simulink model "ENV_old"  (R2024b)
settings: Solver=FixedStepDiscrete  StartTime=0.0  StopTime=1  FixedStep=0.001  RelTol=1e-3  EnableMultiTasking=on
libraries: stm32blockslib x84, canmsglib x40, stm32f4xxblockslib x8, simulink x7
(part 3 of 4)

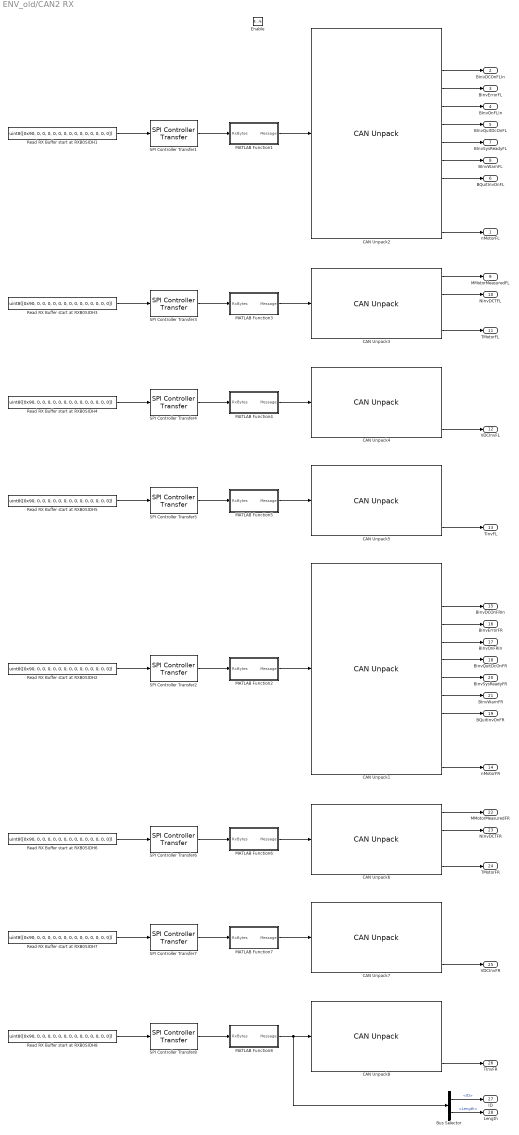
== system ENV_old/CAN2 RX ==
  Enable : EnablePort
  Bus Selector : BusSelector  OutputSignals=ID,Length
  CAN Unpack1 : canmsglib/CAN Unpack  CANdbFile=C:\Users\Will\Desktop\OBR\Embedded\VCUSTM32\Controls\CAN\Inverters\26.06.18_CAN2.dbc  MsgList=INV4_Send_1  MsgName=INV4_Send_1  MsgIDType=Standard (11-bit identifier)  MsgIdentifier=658  MsgLength=8  SignalInfo={'AMK_bDerating','47','1','LE','unsigned','Standard','0','1','0','0','1';'AMK_bReserve','32','8','LE','signed','Standard','0','1','0','-128','127';'BInvDCOnFRIn','44','1','LE','unsigned','Standard','0','1','0','0','1';'BInvErrorFR','41','1','LE','unsigned','Standard','0','1','0','0','1';'BInvOnFRIn','46','1','LE','unsigned','Standard','0','1','0','0','1';'BInvQuitDcOnFR','43','1','LE','unsigned','Standard','0','1','0','0','1';'BInvSysReadyFR','40','1','LE','unsigned','Standard','0','1','0','0','1';'BInvWarnFR','42','1','LE','unsigned','Standard','0','1','0','0','1';'BQuitInvOnFR','45','1','LE','unsigned','Standard','0','1','0','0','1';'Checksum','16','16','LE','unsigned','Standard','0','1','0','0','65535';'Message_Counter','0','16','LE','unsigned','Standard','0','1','0','0','65535';'nMotorFR','48','16','LE','signed','Standard','0','1','0','-32768','32767'}  IDPort=off  TimestampPort=off  ErrorPort=off  RemotePort=off  LengthPort=off  StatusPort=off  ApplyMinMax=off
      settings: LibrarySourceBlock=stmutilitieslib/CAN Unpack  DataFormat=CANdb specified signals
  CAN Unpack2 : canmsglib/CAN Unpack  CANdbFile=C:\Users\Will\Desktop\OBR\Embedded\VCUSTM32\Controls\CAN\Inverters\26.06.18_CAN2.dbc  MsgList=INV2_Send_1  MsgName=INV2_Send_1  MsgIDType=Standard (11-bit identifier)  MsgIdentifier=657  MsgLength=8  SignalInfo={'AMK_bDerating','47','1','LE','unsigned','Standard','0','1','0','0','1';'AMK_bReserve','32','8','LE','signed','Standard','0','1','0','-128','127';'BInvDCOnFLIn','44','1','LE','unsigned','Standard','0','1','0','0','1';'BInvErrorFL','41','1','LE','unsigned','Standard','0','1','0','0','1';'BInvOnFLIn','46','1','LE','unsigned','Standard','0','1','0','0','1';'BInvQuitDcOnFL','43','1','LE','unsigned','Standard','0','1','0','0','1';'BInvSysReadyFL','40','1','LE','unsigned','Standard','0','1','0','0','1';'BInvWarnFL','42','1','LE','unsigned','Standard','0','1','0','0','1';'BQuitInvOnFL','45','1','LE','unsigned','Standard','0','1','0','0','1';'Checksum','16','16','LE','unsigned','Standard','0','1','0','0','65535';'Message_Counter','0','16','LE','unsigned','Standard','0','1','0','0','65535';'nMotorFL','48','16','LE','signed','Standard','0','1','0','-32768','32767'}  IDPort=off  TimestampPort=off  ErrorPort=off  RemotePort=off  LengthPort=off  StatusPort=off  ApplyMinMax=off
      settings: LibrarySourceBlock=stmutilitieslib/CAN Unpack  DataFormat=CANdb specified signals
  CAN Unpack3 : canmsglib/CAN Unpack  CANdbFile=C:\Users\Will\Desktop\OBR\Embedded\VCUSTM32\Controls\CAN\Inverters\26.06.18_CAN2.dbc  MsgList=INV2_Send_2  MsgName=INV2_Send_2  MsgIDType=Standard (11-bit identifier)  MsgIdentifier=659  MsgLength=8  SignalInfo={'MMotorMeasuredFL','16','16','LE','signed','Standard','0','1','0','-32768','32767';'NInvDTCFL','32','16','LE','signed','Standard','0','1','0','-32768','32767';'NInvErrorInfoFL1','48','16','LE','signed','Standard','0','1','0','-32768','32767';'TMotorFL','0','16','LE','signed','Standard','0','0.1','0','-3276.8','3276.7'}  IDPort=off  TimestampPort=off  ErrorPort=off  RemotePort=off  LengthPort=off  StatusPort=off  ApplyMinMax=off
      settings: LibrarySourceBlock=stmutilitieslib/CAN Unpack  DataFormat=CANdb specified signals
  CAN Unpack4 : canmsglib/CAN Unpack  CANdbFile=C:\Users\Will\Desktop\OBR\Embedded\VCUSTM32\Controls\CAN\Inverters\26.06.18_CAN2.dbc  MsgList=INV2_Send_3  MsgName=INV2_Send_3  MsgIDType=Standard (11-bit identifier)  MsgIdentifier=661  MsgLength=8  SignalInfo={'NInvErrorInfoFL2','0','16','LE','signed','Standard','0','1','0','-32768','32767';'NInvErrorInfoFL3','16','16','LE','signed','Standard','0','1','0','-32768','32767';'Raw_Torque_Current','32','16','LE','signed','Standard','0','1','0','-32768','32767';'VDCInvFL','48','16','LE','signed','Standard','0','1','0','-32768','32767'}  IDPort=off  TimestampPort=off  ErrorPort=off  RemotePort=off  LengthPort=off  StatusPort=off  ApplyMinMax=off
      settings: LibrarySourceBlock=stmutilitieslib/CAN Unpack  DataFormat=CANdb specified signals
  CAN Unpack5 : canmsglib/CAN Unpack  CANdbFile=C:\Users\Will\Desktop\OBR\Embedded\VCUSTM32\Controls\CAN\Inverters\26.06.18_CAN2.dbc  MsgList=INV2_Send_4  MsgName=INV2_Send_4  MsgIDType=Standard (11-bit identifier)  MsgIdentifier=663  MsgLength=8  SignalInfo={'Converter_Peak_Current','32','16','LE','signed','Standard','0','1','0','-32768','32767';'Motor_Nomial_Current_IN','48','16','LE','signed','Standard','0','1','0','-32768','32767';'Motor_Peak_Current','16','16','LE','signed','Standard','0','1','0','-32768','32767';'TInvFL','0','16','LE','signed','Standard','0','0.1','0','-3276.8','3276.7'}  IDPort=off  TimestampPort=off  ErrorPort=off  RemotePort=off  LengthPort=off  StatusPort=off  ApplyMinMax=off
      settings: LibrarySourceBlock=stmutilitieslib/CAN Unpack  DataFormat=CANdb specified signals
  CAN Unpack6 : canmsglib/CAN Unpack  CANdbFile=C:\Users\Will\Desktop\OBR\Embedded\VCUSTM32\Controls\CAN\Inverters\26.06.18_CAN2.dbc  MsgList=INV4_Send_2  MsgName=INV4_Send_2  MsgIDType=Standard (11-bit identifier)  MsgIdentifier=660  MsgLength=8  SignalInfo={'MMotorMeasuredFR','16','16','LE','signed','Standard','0','1','0','-32768','32767';'NInvDTCFR','32','16','LE','signed','Standard','0','1','0','-32768','32767';'NInvErrorInfoFR1','48','16','LE','signed','Standard','0','1','0','-32768','32767';'TMotorFR','0','16','LE','signed','Standard','0','0.1','0','-3276.8','3276.7'}  IDPort=off  TimestampPort=off  ErrorPort=off  RemotePort=off  LengthPort=off  StatusPort=off  ApplyMinMax=off
      settings: LibrarySourceBlock=stmutilitieslib/CAN Unpack  DataFormat=CANdb specified signals
  CAN Unpack7 : canmsglib/CAN Unpack  CANdbFile=C:\Users\Will\Desktop\OBR\Embedded\VCUSTM32\Controls\CAN\Inverters\26.06.18_CAN2.dbc  MsgList=INV4_Send_3  MsgName=INV4_Send_3  MsgIDType=Standard (11-bit identifier)  MsgIdentifier=662  MsgLength=8  SignalInfo={'NInvErrorInfoFR2','0','16','LE','signed','Standard','0','1','0','-32768','32767';'NInvErrorInfoFR3','16','16','LE','signed','Standard','0','1','0','-32768','32767';'Raw_Torque_Current','32','16','LE','signed','Standard','0','1','0','-32768','32767';'VDCInvFR','48','16','LE','signed','Standard','0','1','0','-32768','32767'}  IDPort=off  TimestampPort=off  ErrorPort=off  RemotePort=off  LengthPort=off  StatusPort=off  ApplyMinMax=off
      settings: LibrarySourceBlock=stmutilitieslib/CAN Unpack  DataFormat=CANdb specified signals
  CAN Unpack8 : canmsglib/CAN Unpack  CANdbFile=C:\Users\Will\Desktop\OBR\Embedded\VCUSTM32\Controls\CAN\Inverters\26.06.18_CAN2.dbc  MsgList=INV4_Send_4  MsgName=INV4_Send_4  MsgIDType=Standard (11-bit identifier)  MsgIdentifier=664  MsgLength=8  SignalInfo={'Converter_Peak_Current','32','16','LE','signed','Standard','0','1','0','-32768','32767';'Motor_Nomial_Current_IN','48','16','LE','signed','Standard','0','1','0','-32768','32767';'Motor_Peak_Current','16','16','LE','signed','Standard','0','1','0','-32768','32767';'TInvFR','0','16','LE','signed','Standard','0','0.1','0','-3276.8','3276.7'}  IDPort=off  TimestampPort=off  ErrorPort=off  RemotePort=off  LengthPort=off  StatusPort=off  ApplyMinMax=off
      settings: LibrarySourceBlock=stmutilitieslib/CAN Unpack  DataFormat=CANdb specified signals
  MATLAB Function1 : MATLAB Function  TreatAsAtomicUnit=on
  MATLAB Function2 : MATLAB Function  TreatAsAtomicUnit=on
  MATLAB Function3 : MATLAB Function  TreatAsAtomicUnit=on
  MATLAB Function4 : MATLAB Function  TreatAsAtomicUnit=on
  MATLAB Function5 : MATLAB Function  TreatAsAtomicUnit=on
  MATLAB Function6 : MATLAB Function  TreatAsAtomicUnit=on
  MATLAB Function7 : MATLAB Function  TreatAsAtomicUnit=on
  MATLAB Function8 : MATLAB Function  TreatAsAtomicUnit=on
  Read RX Buffer start at RXB0SIDH{1..8} (8 alike) : Constant  Value=uint8([0x90, 0, 0, 0, 0, 0, 0, 0, 0, 0, 0, 0, 0, 0, 0])
  SPI Controller Transfer{1..8} (8 alike) : stm32blockslib/SPI Controller Transfer  Priority=1  SPIModuleSelect=SPI1  ClockPolarity=Low  ClockPhase=1 Edge  SPIModule=uint32(0)  Mode=Master  BusSpeed=uint32(1000000)  FirstBitToTransfer=Most significant bit (MSB)  ClockMode=0  BlockFunction=Transfer  EnableRegisterAddress=off  RegisterAddress=0  OutputDataType=uint8  OutputDataLength=1  OutputStatus=off  BlockingMode=on  Timeout=0.01  DataBits=8  UseCustomSSPin=Explicit GPIO calls  ActiveLowSSPin=Active low  Port_Select=GPIOC  Pin=10
      settings: LibrarySourceBlock=stm32h7xxblockslib/SPI Controller Transfer
  nMotorFL : Outport  OutDataTypeStr=double
  BInvDCOnFLIn : Outport  Port=2  OutDataTypeStr=boolean
  BInvErrorFL : Outport  Port=3  OutDataTypeStr=boolean
  BInvOnFLIn : Outport  Port=4  OutDataTypeStr=boolean
  BInvQuitDcOnFL : Outport  Port=5  OutDataTypeStr=boolean
  BQuitInvOnFL : Outport  Port=6  OutDataTypeStr=boolean
  BInvSysReadyFL : Outport  Port=7  OutDataTypeStr=boolean
  BInvWarnFL : Outport  Port=8  OutDataTypeStr=boolean
  MMotorMeasuredFL : Outport  Port=9  OutDataTypeStr=double
  NInvDCTFL : Outport  Port=10  OutDataTypeStr=double
  TMotorFL : Outport  Port=11  OutDataTypeStr=double
  VDCInvFL : Outport  Port=12  OutDataTypeStr=double
  TInvFL : Outport  Port=13  OutDataTypeStr=double
  nMotorFR : Outport  Port=14  OutDataTypeStr=double
  BInvDCOnFRIn : Outport  Port=15  OutDataTypeStr=boolean
  BInvErrorFR : Outport  Port=16  OutDataTypeStr=boolean
  BInvOnFRIn : Outport  Port=17  OutDataTypeStr=boolean
  BInvQuitDcOnFR : Outport  Port=18  OutDataTypeStr=boolean
  BQuitInvOnFR : Outport  Port=19  OutDataTypeStr=boolean
  BInvSysReadyFR : Outport  Port=20  OutDataTypeStr=boolean
  BInvWarnFR : Outport  Port=21  OutDataTypeStr=boolean
  MMotorMeasuredFR : Outport  Port=22  OutDataTypeStr=double
  NInvDCTFR : Outport  Port=23  OutDataTypeStr=double
  TMotorFR : Outport  Port=24  OutDataTypeStr=double
  VDCInvFR : Outport  Port=25  OutDataTypeStr=double
  TInvFR : Outport  Port=26  OutDataTypeStr=double
  ID : Outport  Port=27
  Length : Outport  Port=28
  wires:
  Read RX Buffer start at RXB0SIDH1/1 -> SPI Controller Transfer1/1
  SPI Controller Transfer1/1 -> MATLAB Function1/1(RxBytes)
  MATLAB Function1/1(Message) -> CAN Unpack2/1
  CAN Unpack2/3 -> BInvDCOnFLIn/1
  CAN Unpack2/4 -> BInvErrorFL/1
  CAN Unpack2/5 -> BInvOnFLIn/1
  CAN Unpack2/6 -> BInvQuitDcOnFL/1
  CAN Unpack2/9 -> BQuitInvOnFL/1
  CAN Unpack2/8 -> BInvWarnFL/1
  CAN Unpack2/7 -> BInvSysReadyFL/1
  CAN Unpack2/12 -> nMotorFL/1
  CAN Unpack3/4 -> TMotorFL/1
  MATLAB Function3/1(Message) -> CAN Unpack3/1
  SPI Controller Transfer3/1 -> MATLAB Function3/1(RxBytes)
  Read RX Buffer start at RXB0SIDH3/1 -> SPI Controller Transfer3/1
  CAN Unpack3/1 -> MMotorMeasuredFL/1
  CAN Unpack3/2 -> NInvDCTFL/1
  CAN Unpack4/4 -> VDCInvFL/1
  SPI Controller Transfer4/1 -> MATLAB Function4/1(RxBytes)
  MATLAB Function4/1(Message) -> CAN Unpack4/1
  Read RX Buffer start at RXB0SIDH4/1 -> SPI Controller Transfer4/1
  SPI Controller Transfer5/1 -> MATLAB Function5/1(RxBytes)
  CAN Unpack5/4 -> TInvFL/1
  Read RX Buffer start at RXB0SIDH5/1 -> SPI Controller Transfer5/1
  MATLAB Function5/1(Message) -> CAN Unpack5/1
  MATLAB Function8/1(Message) -> Bus Selector/1, CAN Unpack8/1
  Bus Selector/2 -> Length/1  "<Length>"
  Bus Selector/1 -> ID/1  "<ID>"
  CAN Unpack1/6 -> BInvQuitDcOnFR/1
  CAN Unpack1/3 -> BInvDCOnFRIn/1
  CAN Unpack6/4 -> TMotorFR/1
  CAN Unpack1/5 -> BInvOnFRIn/1
  SPI Controller Transfer2/1 -> MATLAB Function2/1(RxBytes)
  MATLAB Function2/1(Message) -> CAN Unpack1/1
  SPI Controller Transfer8/1 -> MATLAB Function8/1(RxBytes)
  CAN Unpack1/8 -> BInvWarnFR/1
  CAN Unpack6/1 -> MMotorMeasuredFR/1
  CAN Unpack1/12 -> nMotorFR/1
  CAN Unpack1/4 -> BInvErrorFR/1
  CAN Unpack1/7 -> BInvSysReadyFR/1
  CAN Unpack1/9 -> BQuitInvOnFR/1
  Read RX Buffer start at RXB0SIDH2/1 -> SPI Controller Transfer2/1
  SPI Controller Transfer7/1 -> MATLAB Function7/1(RxBytes)
  Read RX Buffer start at RXB0SIDH8/1 -> SPI Controller Transfer8/1
  MATLAB Function6/1(Message) -> CAN Unpack6/1
  Read RX Buffer start at RXB0SIDH7/1 -> SPI Controller Transfer7/1
  CAN Unpack6/2 -> NInvDCTFR/1
  SPI Controller Transfer6/1 -> MATLAB Function6/1(RxBytes)
  MATLAB Function7/1(Message) -> CAN Unpack7/1
  Read RX Buffer start at RXB0SIDH6/1 -> SPI Controller Transfer6/1
  CAN Unpack7/4 -> VDCInvFR/1
  CAN Unpack8/4 -> TInvFR/1

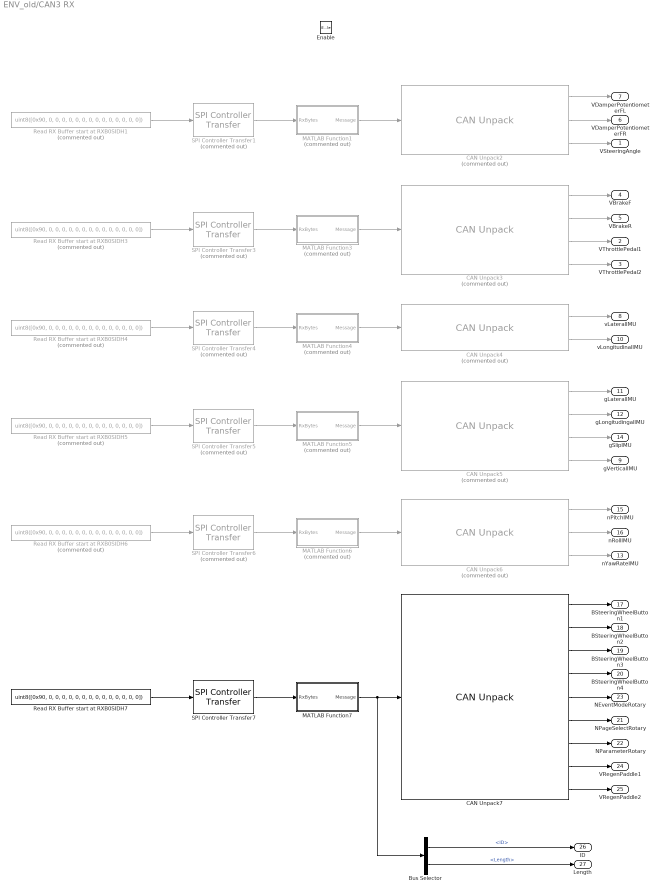
== system ENV_old/CAN3 RX ==
  Enable : EnablePort
  Bus Selector : BusSelector  OutputSignals=ID,Length
  CAN Unpack2 : canmsglib/CAN Unpack  Commented=on  CANdbFile=C:\Users\oxbro\Documents\STM32CustomProjects\VCUSTM32\OBR26_Controls_30-7-26\CAN\CAN3\CAN3_03.08.26.dbc  MsgList=(none)  MsgName=DDU7_SteerDamper  MsgIDType=Standard (11-bit identifier)  MsgIdentifier=257  MsgLength=8  SignalInfo={'VDamperPotentiometerFL','16','13','LE','unsigned','Standard','0','1','0','0','8191';'VDamperPotentiometerFR','29','13','LE','unsigned','Standard','0','1','0','0','8191';'VSteeringAngle','0','13','LE','unsigned','Standard','0','1','0','0','8191'}  IDPort=off  TimestampPort=off  ErrorPort=off  RemotePort=off  LengthPort=off  StatusPort=off  ApplyMinMax=off
      settings: LibrarySourceBlock=stmutilitieslib/CAN Unpack  DataFormat=CANdb specified signals
  CAN Unpack3 : canmsglib/CAN Unpack  Commented=on  CANdbFile=C:\Users\oxbro\Documents\STM32CustomProjects\VCUSTM32\OBR26_Controls_30-7-26\CAN\CAN3\CAN3_03.08.26.dbc  MsgList=(none)  MsgName=DDU7_ThrBrake  MsgIDType=Standard (11-bit identifier)  MsgIdentifier=256  MsgLength=8  SignalInfo={'VBrakeF','0','16','LE','unsigned','Standard','0','1','0','0','3276.75';'VBrakeR','16','16','LE','unsigned','Standard','0','1','0','0','65535';'VThrottlePedal1','32','16','LE','unsigned','Standard','0','1','0','0','65535';'VThrottlePedal2','48','16','LE','unsigned','Standard','0','1','0','0','65535'}  IDPort=off  TimestampPort=off  ErrorPort=off  RemotePort=off  LengthPort=off  StatusPort=off  ApplyMinMax=off
      settings: LibrarySourceBlock=stmutilitieslib/CAN Unpack  DataFormat=CANdb specified signals
  CAN Unpack4 : canmsglib/CAN Unpack  Commented=on  CANdbFile=C:\Users\oxbro\Documents\STM32CustomProjects\VCUSTM32\OBR26_Controls_30-7-26\CAN\CAN3\CAN3_03.08.26.dbc  MsgList=(none)  MsgName=IMU_0x604  MsgIDType=Standard (11-bit identifier)  MsgIdentifier=1540  MsgLength=8  SignalInfo={'vLateralIMU','16','16','LE','signed','Standard','0','0.01','0','-327.68','327.67';'vLongitudinalIMU','0','16','LE','signed','Standard','0','0.01','0','-327.68','327.67'}  IDPort=off  TimestampPort=off  ErrorPort=off  RemotePort=off  LengthPort=off  StatusPort=off  ApplyMinMax=off
      settings: LibrarySourceBlock=stmutilitieslib/CAN Unpack  DataFormat=CANdb specified signals
  CAN Unpack5 : canmsglib/CAN Unpack  Commented=on  CANdbFile=C:\Users\oxbro\Documents\STM32CustomProjects\VCUSTM32\OBR26_Controls_30-7-26\CAN\CAN3\CAN3_03.08.26.dbc  MsgList=(none)  MsgName=IMU_0x606  MsgIDType=Standard (11-bit identifier)  MsgIdentifier=1542  MsgLength=8  SignalInfo={'gLateralIMU','16','16','LE','signed','Standard','0','0.01','0','-327.68','327.67';'gLongitudinalIMU','0','16','LE','signed','Standard','0','0.01','0','-327.68','327.67';'gSlipIMU','48','16','LE','signed','Standard','0','0.01','0','-327.68','327.67';'gVerticalIMU','32','16','LE','signed','Standard','0','0.01','0','-327.68','327.67'}  IDPort=off  TimestampPort=off  ErrorPort=off  RemotePort=off  LengthPort=off  StatusPort=off  ApplyMinMax=off
      settings: LibrarySourceBlock=stmutilitieslib/CAN Unpack  DataFormat=CANdb specified signals
  CAN Unpack6 : canmsglib/CAN Unpack  Commented=on  CANdbFile=C:\Users\oxbro\Documents\STM32CustomProjects\VCUSTM32\OBR26_Controls_30-7-26\CAN\CAN3\CAN3_03.08.26.dbc  MsgList=(none)  MsgName=IMU_0x609  MsgIDType=Standard (11-bit identifier)  MsgIdentifier=1545  MsgLength=8  SignalInfo={'nPitchIMU','16','16','LE','signed','Standard','0','0.01','0','-327.68','327.67';'nRollIMU','0','16','LE','signed','Standard','0','0.01','0','-327.68','327.67';'nYawRateIMU','32','16','LE','signed','Standard','0','0.01','0','-327.68','327.67'}  IDPort=off  TimestampPort=off  ErrorPort=off  RemotePort=off  LengthPort=off  StatusPort=off  ApplyMinMax=off
      settings: LibrarySourceBlock=stmutilitieslib/CAN Unpack  DataFormat=CANdb specified signals
  CAN Unpack7 : canmsglib/CAN Unpack  CANdbFile=C:\Users\oxbro\Documents\STM32CustomProjects\VCUSTM32\OBR26_Controls_30-7-26\CAN\CAN3\CAN3_03.08.26.dbc  MsgList=STW_0x1FB  MsgName=STW_0x1FB  MsgIDType=Standard (11-bit identifier)  MsgIdentifier=507  MsgLength=6  SignalInfo={'BSteeringWheelButton1','0','1','LE','unsigned','Standard','0','1','0','0','1';'BSteeringWheelButton2','1','1','LE','unsigned','Standard','0','1','0','0','1';'BSteeringWheelButton3','2','1','LE','unsigned','Standard','0','1','0','0','1';'BSteeringWheelButton4','3','1','LE','unsigned','Standard','0','1','0','0','1';'NEventModeRotary','20','8','LE','unsigned','Standard','0','1','1','1','16';'NPageSelectRotary','4','8','LE','unsigned','Standard','0','1','1','1','16';'NParameterRotary','12','8','LE','unsigned','Standard','0','1','1','1','16';'VRegenPaddle1','28','8','LE','unsigned','Standard','0','0.0129','0','0','3.2895';'VRegenPaddle2','36','8','LE','unsigned','Standard','0','0.0129','0','0','3.2895'}  IDPort=off  TimestampPort=off  ErrorPort=off  RemotePort=off  LengthPort=off  StatusPort=off  ApplyMinMax=off
      settings: LibrarySourceBlock=stmutilitieslib/CAN Unpack  DataFormat=CANdb specified signals
  MATLAB Function1 : MATLAB Function  Commented=on  TreatAsAtomicUnit=on
  MATLAB Function3 : MATLAB Function  Commented=on  TreatAsAtomicUnit=on
  MATLAB Function4 : MATLAB Function  Commented=on  TreatAsAtomicUnit=on
  MATLAB Function5 : MATLAB Function  Commented=on  TreatAsAtomicUnit=on
  MATLAB Function6 : MATLAB Function  Commented=on  TreatAsAtomicUnit=on
  MATLAB Function7 : MATLAB Function  TreatAsAtomicUnit=on
  Read RX Buffer start at RXB0SIDH{1,3..6} (5 alike) : Constant  Commented=on  Value=uint8([0x90, 0, 0, 0, 0, 0, 0, 0, 0, 0, 0, 0, 0, 0, 0])
  Read RX Buffer start at RXB0SIDH7 : Constant  Value=uint8([0x90, 0, 0, 0, 0, 0, 0, 0, 0, 0, 0, 0, 0, 0, 0])
  SPI Controller Transfer{1,3..6} (5 alike) : stm32blockslib/SPI Controller Transfer  Priority=1  Commented=on  SPIModuleSelect=SPI1  ClockPolarity=Low  ClockPhase=1 Edge  SPIModule=uint32(0)  Mode=Master  BusSpeed=uint32(1000000)  FirstBitToTransfer=Most significant bit (MSB)  ClockMode=0  BlockFunction=Transfer  EnableRegisterAddress=off  RegisterAddress=0  OutputDataType=uint8  OutputDataLength=1  OutputStatus=off  BlockingMode=on  Timeout=0.01  DataBits=8  UseCustomSSPin=Explicit GPIO calls  ActiveLowSSPin=Active low  Port_Select=GPIOA  Pin=1
      settings: LibrarySourceBlock=stm32h7xxblockslib/SPI Controller Transfer
  SPI Controller Transfer7 : stm32blockslib/SPI Controller Transfer  Priority=1  SPIModuleSelect=SPI1  ClockPolarity=Low  ClockPhase=1 Edge  SPIModule=uint32(0)  Mode=Master  BusSpeed=uint32(1000000)  FirstBitToTransfer=Most significant bit (MSB)  ClockMode=0  BlockFunction=Transfer  EnableRegisterAddress=off  RegisterAddress=0  OutputDataType=uint8  OutputDataLength=1  OutputStatus=off  BlockingMode=on  Timeout=0.01  DataBits=8  UseCustomSSPin=Explicit GPIO calls  ActiveLowSSPin=Active low  Port_Select=GPIOA  Pin=1
      settings: LibrarySourceBlock=stm32h7xxblockslib/SPI Controller Transfer
  VSteeringAngle : Outport  OutDataTypeStr=double
  VThrottlePedal1 : Outport  Port=2  OutDataTypeStr=double
  VThrottlePedal2 : Outport  Port=3  OutDataTypeStr=double
  VBrakeF : Outport  Port=4  OutDataTypeStr=double
  VBrakeR : Outport  Port=5  OutDataTypeStr=double
  VDamperPotentiometerFR : Outport  Port=6  OutDataTypeStr=double
  VDamperPotentiometerFL : Outport  Port=7  OutDataTypeStr=double
  vLateralIMU : Outport  Port=8  OutDataTypeStr=double
  gVerticalIMU : Outport  Port=9  OutDataTypeStr=double
  vLongitudinalIMU : Outport  Port=10  OutDataTypeStr=double
  gLateralIMU : Outport  Port=11  OutDataTypeStr=double
  gLongitudingalIMU : Outport  Port=12  OutDataTypeStr=double
  nYawRateIMU : Outport  Port=13  OutDataTypeStr=double
  gSlipIMU : Outport  Port=14  OutDataTypeStr=double
  nPitchIMU : Outport  Port=15  OutDataTypeStr=double
  nRollIMU : Outport  Port=16  OutDataTypeStr=double
  BSteeringWheelButton1 : Outport  Port=17  OutDataTypeStr=boolean
  BSteeringWheelButton2 : Outport  Port=18  OutDataTypeStr=boolean
  BSteeringWheelButton3 : Outport  Port=19  OutDataTypeStr=boolean
  BSteeringWheelButton4 : Outport  Port=20  OutDataTypeStr=boolean
  NPageSelectRotary : Outport  Port=21  OutDataTypeStr=double
  NParameterRotary : Outport  Port=22  OutDataTypeStr=double
  NEventModeRotary : Outport  Port=23  OutDataTypeStr=double
  VRegenPaddle1 : Outport  Port=24  OutDataTypeStr=double
  VRegenPaddle2 : Outport  Port=25  OutDataTypeStr=double
  ID : Outport  Port=26
  Length : Outport  Port=27
  wires:
  Bus Selector/1 -> ID/1  "<ID>"
  Bus Selector/2 -> Length/1  "<Length>"
  CAN Unpack4/1 -> vLateralIMU/1
  CAN Unpack7/5 -> NEventModeRotary/1
  CAN Unpack7/3 -> BSteeringWheelButton3/1
  CAN Unpack2/1 -> VDamperPotentiometerFL/1
  CAN Unpack2/2 -> VDamperPotentiometerFR/1
  CAN Unpack5/4 -> gVerticalIMU/1
  CAN Unpack3/3 -> VThrottlePedal1/1
  CAN Unpack2/3 -> VSteeringAngle/1
  CAN Unpack6/2 -> nRollIMU/1
  CAN Unpack7/6 -> NPageSelectRotary/1
  CAN Unpack7/1 -> BSteeringWheelButton1/1
  CAN Unpack6/3 -> nYawRateIMU/1
  CAN Unpack3/1 -> VBrakeF/1
  CAN Unpack5/2 -> gLongitudingalIMU/1
  CAN Unpack7/9 -> VRegenPaddle2/1
  CAN Unpack7/7 -> NParameterRotary/1
  CAN Unpack7/2 -> BSteeringWheelButton2/1
  CAN Unpack3/4 -> VThrottlePedal2/1
  CAN Unpack3/2 -> VBrakeR/1
  CAN Unpack7/8 -> VRegenPaddle1/1
  CAN Unpack6/1 -> nPitchIMU/1
  CAN Unpack5/3 -> gSlipIMU/1
  CAN Unpack7/4 -> BSteeringWheelButton4/1
  CAN Unpack4/2 -> vLongitudinalIMU/1
  CAN Unpack5/1 -> gLateralIMU/1
  Read RX Buffer start at RXB0SIDH1/1 -> SPI Controller Transfer1/1
  SPI Controller Transfer1/1 -> MATLAB Function1/1(RxBytes)
  MATLAB Function1/1(Message) -> CAN Unpack2/1
  MATLAB Function3/1(Message) -> CAN Unpack3/1
  Read RX Buffer start at RXB0SIDH3/1 -> SPI Controller Transfer3/1
  SPI Controller Transfer3/1 -> MATLAB Function3/1(RxBytes)
  MATLAB Function4/1(Message) -> CAN Unpack4/1
  Read RX Buffer start at RXB0SIDH4/1 -> SPI Controller Transfer4/1
  SPI Controller Transfer4/1 -> MATLAB Function4/1(RxBytes)
  Read RX Buffer start at RXB0SIDH5/1 -> SPI Controller Transfer5/1
  SPI Controller Transfer5/1 -> MATLAB Function5/1(RxBytes)
  MATLAB Function5/1(Message) -> CAN Unpack5/1
  Read RX Buffer start at RXB0SIDH6/1 -> SPI Controller Transfer6/1
  SPI Controller Transfer6/1 -> MATLAB Function6/1(RxBytes)
  MATLAB Function6/1(Message) -> CAN Unpack6/1
  Read RX Buffer start at RXB0SIDH7/1 -> SPI Controller Transfer7/1
  SPI Controller Transfer7/1 -> MATLAB Function7/1(RxBytes)
  MATLAB Function7/1(Message) -> Bus Selector/1, CAN Unpack7/1

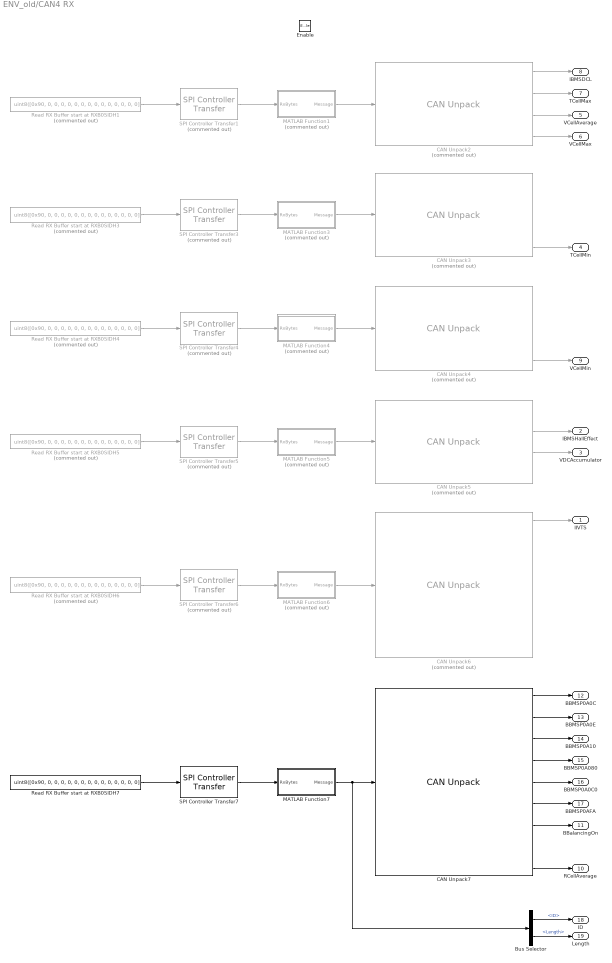
== system ENV_old/CAN4 RX ==
  Enable : EnablePort
  Bus Selector : BusSelector  OutputSignals=ID,Length
  CAN Unpack2 : canmsglib/CAN Unpack  Commented=on  CANdbFile=C:\Users\Will\Desktop\OBR\Embedded\VCUSTM32\Controls\CAN\BMS\26.06.18_CAN4.dbc  MsgList=MSGID_0X6B2  MsgName=MSGID_0X6B2  MsgIDType=Standard (11-bit identifier)  MsgIdentifier=1714  MsgLength=8  SignalInfo={'IBMSDCL','48','16','LE','unsigned','Standard','0','1','0','0','65535';'TCellMax','40','16','BE','signed','Standard','0','1','0','80','32767';'VCellAverage','8','16','BE','unsigned','Standard','0','1e-08','0','0','0.00065535';'VCellMax','24','16','BE','unsigned','Standard','0','0.0001','0','0','6.5535'}  IDPort=off  TimestampPort=off  ErrorPort=off  RemotePort=off  LengthPort=off  StatusPort=off  ApplyMinMax=off
      settings: LibrarySourceBlock=stmutilitieslib/CAN Unpack  DataFormat=CANdb specified signals
  CAN Unpack3 : canmsglib/CAN Unpack  Commented=on  CANdbFile=C:\Users\Will\Desktop\OBR\Embedded\VCUSTM32\Controls\CAN\BMS\26.06.18_CAN4.dbc  MsgList=MSGID_0X6B1  MsgName=MSGID_0X6B1  MsgIDType=Standard (11-bit identifier)  MsgIdentifier=1713  MsgLength=8  SignalInfo={'DTC_Flags_1','16','16','LE','unsigned','Standard','0','1','0','0','65535';'DTC_Flags_2','40','16','BE','unsigned','Standard','0','1','0','0','65535';'Pack_SOC','8','16','BE','unsigned','Standard','0','0.5','0','0','32767.5';'TCellMin','56','16','BE','signed','Standard','0','1','0','80','32767'}  IDPort=off  TimestampPort=off  ErrorPort=off  RemotePort=off  LengthPort=off  StatusPort=off  ApplyMinMax=off
      settings: LibrarySourceBlock=stmutilitieslib/CAN Unpack  DataFormat=CANdb specified signals
  CAN Unpack4 : canmsglib/CAN Unpack  Commented=on  CANdbFile=C:\Users\Will\Desktop\OBR\Embedded\VCUSTM32\Controls\CAN\BMS\26.06.18_CAN4.dbc  MsgList=MSGID_0X6B3  MsgName=MSGID_0X6B3  MsgIDType=Standard (11-bit identifier)  MsgIdentifier=1715  MsgLength=8  SignalInfo={'High_Cell_Resistance','8','16','BE','unsigned','Standard','0','0.01','0','0','655';'Maximum_Cell_Voltage','40','16','BE','unsigned','Standard','0','0.0001','0','0','6.5535';'Minimum_Cell_Voltage','56','16','BE','unsigned','Standard','0','0.0001','0','0','6.5535';'VCellMin','24','16','BE','unsigned','Standard','0','0.0001','0','0','6.5535'}  IDPort=off  TimestampPort=off  ErrorPort=off  RemotePort=off  LengthPort=off  StatusPort=off  ApplyMinMax=off
      settings: LibrarySourceBlock=stmutilitieslib/CAN Unpack  DataFormat=CANdb specified signals
  CAN Unpack5 : canmsglib/CAN Unpack  Commented=on  CANdbFile=C:\Users\Will\Desktop\OBR\Embedded\VCUSTM32\Controls\CAN\BMS\26.06.18_CAN4.dbc  MsgList=MSGID_0X6B0  MsgName=MSGID_0X6B0  MsgIDType=Standard (11-bit identifier)  MsgIdentifier=1712  MsgLength=8  SignalInfo={'CRC_Checksum','48','16','LE','unsigned','Standard','0','1','0','0','65535';'IBMSHallEffect','32','16','LE','signed','Standard','0','1','0','32767','32767';'VDCAccumulator','16','16','LE','unsigned','Standard','0','1','0','0','65535';'VDCAccumulator_NOT','8','16','BE','unsigned','Standard','0','0.1','0','0','6553.5'}  IDPort=off  TimestampPort=off  ErrorPort=off  RemotePort=off  LengthPort=off  StatusPort=off  ApplyMinMax=off
      settings: LibrarySourceBlock=stmutilitieslib/CAN Unpack  DataFormat=CANdb specified signals
  CAN Unpack6 : canmsglib/CAN Unpack  Commented=on  CANdbFile=C:\Users\Will\Desktop\OBR\Embedded\VCUSTM32\Controls\CAN\BMS\26.06.18_CAN4.dbc  MsgList=IVT_Msg_Result_I  MsgName=IVT_Msg_Result_I  MsgIDType=Standard (11-bit identifier)  MsgIdentifier=1313  MsgLength=6  SignalInfo={'IIVTS','40','32','BE','signed','Standard','0','1','0','-2147483648','2147483647';'IVT_ID_Result_I','0','8','BE','unsigned','Standard','0','1','0','0','255';'IVT_MsgCount_Result_I','8','4','BE','unsigned','Standard','0','1','0','0','15';'IVT_Result_I_Channel_Error','13','1','BE','unsigned','Standard','0','1','0','0','1';'IVT_Result_I_Measurement_Error','14','1','BE','unsigned','Standard','0','1','0','0','1';'IVT_Result_I_OCS','12','1','BE','unsigned','Standard','0','1','0','0','1';'IVT_Result_I_System_Error','15','1','BE','unsigned','Standard','0','1','0','0','1'}  IDPort=off  TimestampPort=off  ErrorPort=off  RemotePort=off  LengthPort=off  StatusPort=off  ApplyMinMax=off
      settings: LibrarySourceBlock=stmutilitieslib/CAN Unpack  DataFormat=CANdb specified signals
  CAN Unpack7 : canmsglib/CAN Unpack  CANdbFile=C:\Users\Will\Desktop\OBR\Embedded\VCUSTM32\Controls\CAN\BMS\26.06.18_CAN4.dbc  MsgList=MSGID_0X6B4  MsgName=MSGID_0X6B4  MsgIDType=Standard (11-bit identifier)  MsgIdentifier=1716  MsgLength=8  SignalInfo={'BBMSP0A0C','33','1','LE','unsigned','Standard','0','1','0','0','1';'BBMSP0A0E','34','1','LE','unsigned','Standard','0','1','0','0','1';'BBMSP0A10','35','1','LE','unsigned','Standard','0','1','0','0','1';'BBMSP0A80','36','1','LE','unsigned','Standard','0','1','0','0','1';'BBMSP0AC0','37','1','LE','unsigned','Standard','0','1','0','0','1';'BBMSP0AFA','38','1','LE','unsigned','Standard','0','1','0','0','1';'BBalancingOn','32','1','LE','unsigned','Standard','0','1','0','0','1';'Blank','56','8','LE','unsigned','Standard','0','1','0','0','255';'RCellAverage','8','16','BE','unsigned','Standard','0','0.01','0','0','655'}  IDPort=off  TimestampPort=off  ErrorPort=off  RemotePort=off  LengthPort=off  StatusPort=off  ApplyMinMax=off
      settings: LibrarySourceBlock=stmutilitieslib/CAN Unpack  DataFormat=CANdb specified signals
  MATLAB Function1 : MATLAB Function  Commented=on  TreatAsAtomicUnit=on
  MATLAB Function3 : MATLAB Function  Commented=on  TreatAsAtomicUnit=on
  MATLAB Function4 : MATLAB Function  Commented=on  TreatAsAtomicUnit=on
  MATLAB Function5 : MATLAB Function  Commented=on  TreatAsAtomicUnit=on
  MATLAB Function6 : MATLAB Function  Commented=on  TreatAsAtomicUnit=on
  MATLAB Function7 : MATLAB Function  TreatAsAtomicUnit=on
  Read RX Buffer start at RXB0SIDH{1,3..6} (5 alike) : Constant  Commented=on  Value=uint8([0x90, 0, 0, 0, 0, 0, 0, 0, 0, 0, 0, 0, 0, 0, 0])
  Read RX Buffer start at RXB0SIDH7 : Constant  Value=uint8([0x90, 0, 0, 0, 0, 0, 0, 0, 0, 0, 0, 0, 0, 0, 0])
  SPI Controller Transfer{1,3..6} (5 alike) : stm32blockslib/SPI Controller Transfer  Priority=1  Commented=on  SPIModuleSelect=SPI1  ClockPolarity=Low  ClockPhase=1 Edge  SPIModule=uint32(0)  Mode=Master  BusSpeed=uint32(1000000)  FirstBitToTransfer=Most significant bit (MSB)  ClockMode=0  BlockFunction=Transfer  EnableRegisterAddress=off  RegisterAddress=0  OutputDataType=uint8  OutputDataLength=1  OutputStatus=off  BlockingMode=on  Timeout=0.01  DataBits=8  UseCustomSSPin=Explicit GPIO calls  ActiveLowSSPin=Active low  Port_Select=GPIOC  Pin=5
      settings: LibrarySourceBlock=stm32h7xxblockslib/SPI Controller Transfer
  SPI Controller Transfer7 : stm32blockslib/SPI Controller Transfer  Priority=1  SPIModuleSelect=SPI1  ClockPolarity=Low  ClockPhase=1 Edge  SPIModule=uint32(0)  Mode=Master  BusSpeed=uint32(1000000)  FirstBitToTransfer=Most significant bit (MSB)  ClockMode=0  BlockFunction=Transfer  EnableRegisterAddress=off  RegisterAddress=0  OutputDataType=uint8  OutputDataLength=1  OutputStatus=off  BlockingMode=on  Timeout=0.01  DataBits=8  UseCustomSSPin=Explicit GPIO calls  ActiveLowSSPin=Active low  Port_Select=GPIOC  Pin=5
      settings: LibrarySourceBlock=stm32h7xxblockslib/SPI Controller Transfer
  IIVTS : Outport  OutDataTypeStr=double
  IBMSHallEffect : Outport  Port=2  OutDataTypeStr=double
  VDCAccumulator : Outport  Port=3  OutDataTypeStr=double
  TCellMin : Outport  Port=4  OutDataTypeStr=double
  VCellAverage : Outport  Port=5  OutDataTypeStr=double
  VCellMax : Outport  Port=6  OutDataTypeStr=double
  TCellMax : Outport  Port=7  OutDataTypeStr=double
  IBMSDCL : Outport  Port=8  OutDataTypeStr=double
  VCellMin : Outport  Port=9  OutDataTypeStr=double
  RCellAverage : Outport  Port=10  OutDataTypeStr=double
  BBalancingOn : Outport  Port=11  OutDataTypeStr=boolean
  BBMSP0A0C : Outport  Port=12  OutDataTypeStr=boolean
  BBMSP0A0E : Outport  Port=13  OutDataTypeStr=boolean
  BBMSP0A10 : Outport  Port=14  OutDataTypeStr=boolean
  BBMSP0A080 : Outport  Port=15  OutDataTypeStr=boolean
  BBMSP0A0C0 : Outport  Port=16  OutDataTypeStr=boolean
  BBMSP0AFA : Outport  Port=17  OutDataTypeStr=boolean
  ID : Outport  Port=18
  Length : Outport  Port=19
  wires:
  Bus Selector/1 -> ID/1  "<ID>"
  Bus Selector/2 -> Length/1  "<Length>"
  CAN Unpack2/1 -> IBMSDCL/1
  CAN Unpack2/2 -> TCellMax/1
  CAN Unpack2/3 -> VCellAverage/1
  CAN Unpack5/2 -> IBMSHallEffect/1
  CAN Unpack6/1 -> IIVTS/1
  CAN Unpack5/3 -> VDCAccumulator/1
  Read RX Buffer start at RXB0SIDH1/1 -> SPI Controller Transfer1/1
  SPI Controller Transfer1/1 -> MATLAB Function1/1(RxBytes)
  MATLAB Function1/1(Message) -> CAN Unpack2/1
  MATLAB Function3/1(Message) -> CAN Unpack3/1
  Read RX Buffer start at RXB0SIDH3/1 -> SPI Controller Transfer3/1
  SPI Controller Transfer3/1 -> MATLAB Function3/1(RxBytes)
  MATLAB Function4/1(Message) -> CAN Unpack4/1
  Read RX Buffer start at RXB0SIDH4/1 -> SPI Controller Transfer4/1
  SPI Controller Transfer4/1 -> MATLAB Function4/1(RxBytes)
  Read RX Buffer start at RXB0SIDH5/1 -> SPI Controller Transfer5/1
  SPI Controller Transfer5/1 -> MATLAB Function5/1(RxBytes)
  MATLAB Function5/1(Message) -> CAN Unpack5/1
  Read RX Buffer start at RXB0SIDH6/1 -> SPI Controller Transfer6/1
  SPI Controller Transfer6/1 -> MATLAB Function6/1(RxBytes)
  MATLAB Function6/1(Message) -> CAN Unpack6/1
  Read RX Buffer start at RXB0SIDH7/1 -> SPI Controller Transfer7/1
  SPI Controller Transfer7/1 -> MATLAB Function7/1(RxBytes)
  MATLAB Function7/1(Message) -> Bus Selector/1, CAN Unpack7/1
  CAN Unpack3/4 -> TCellMin/1
  CAN Unpack2/4 -> VCellMax/1
  CAN Unpack4/4 -> VCellMin/1
  CAN Unpack7/2 -> BBMSP0A0E/1
  CAN Unpack7/3 -> BBMSP0A10/1
  CAN Unpack7/1 -> BBMSP0A0C/1
  CAN Unpack7/9 -> RCellAverage/1
  CAN Unpack7/7 -> BBalancingOn/1
  CAN Unpack7/6 -> BBMSP0AFA/1
  CAN Unpack7/5 -> BBMSP0A0C0/1
  CAN Unpack7/4 -> BBMSP0A080/1

== system ENV_old/Initialize CAN1 ==
  Detect Increase : simulink/Logic and Bit Operations/Detect Increase  vinit=0.0  OutDataTypeStr=boolean
  MCPInit : Subsystem  TreatAsAtomicUnit=on
  Step1 : Step
  Step2 : Step
  Unit Delay : UnitDelay  SampleTime=-1  HasFrameUpgradeWarning=on
  MCPInitialized : Outport
  wires:
  Step1/1 -> Detect Increase/1
  Detect Increase/1 -> MCPInit/Enable
  Step2/1 -> Unit Delay/1
  Unit Delay/1 -> MCPInitialized/1

== system ENV_old/Initialize CAN2 ==
  Detect Increase : simulink/Logic and Bit Operations/Detect Increase  vinit=0.0  OutDataTypeStr=boolean
  MCPInit : Subsystem  TreatAsAtomicUnit=on
  Step1 : Step
  Step2 : Step
  Unit Delay : UnitDelay  SampleTime=-1  HasFrameUpgradeWarning=on
  Unit Delay1 : UnitDelay  SampleTime=-1  HasFrameUpgradeWarning=on
  Unit Delay2 : UnitDelay  SampleTime=-1  HasFrameUpgradeWarning=on
  MCPInitialized : Outport
  wires:
  Step1/1 -> Unit Delay1/1
  Detect Increase/1 -> MCPInit/Enable
  Step2/1 -> Unit Delay/1
  Unit Delay/1 -> Unit Delay2/1
  Unit Delay1/1 -> Detect Increase/1
  Unit Delay2/1 -> MCPInitialized/1

== system ENV_old/Initialize CAN3 ==
  Detect Increase : simulink/Logic and Bit Operations/Detect Increase  vinit=0.0  OutDataTypeStr=boolean
  Initialize : Subsystem  TreatAsAtomicUnit=on
  MCPInit : Subsystem  TreatAsAtomicUnit=on
  Step1 : Step
  Step2 : Step
  Unit Delay{1..5} (5 alike) : UnitDelay  SampleTime=-1  HasFrameUpgradeWarning=on
  MCPInitialized : Outport
  wires:
  Initialize/1(MCPInitialized) -> MCPInitialized/1
  Detect Increase/1 -> MCPInit/Enable
  Step1/1 -> Unit Delay3/1
  Step2/1 -> Unit Delay1/1
  Unit Delay3/1 -> Unit Delay4/1
  Unit Delay4/1 -> Detect Increase/1
  Unit Delay1/1 -> Unit Delay2/1
  Unit Delay2/1 -> Unit Delay5/1
  Unit Delay5/1 -> Initialize/Enable

== system ENV_old/Initialize CAN4 ==
  Detect Increase : simulink/Logic and Bit Operations/Detect Increase  vinit=0.0  OutDataTypeStr=boolean
  MCPInit : Subsystem  TreatAsAtomicUnit=on
  Step1 : Step
  Step2 : Step
  Unit Delay{1..7} (7 alike) : UnitDelay  SampleTime=-1  HasFrameUpgradeWarning=on
  MCPInitialized : Outport
  wires:
  Step1/1 -> Unit Delay3/1
  Detect Increase/1 -> MCPInit/Enable
  Step2/1 -> Unit Delay7/1
  Unit Delay3/1 -> Unit Delay1/1
  Unit Delay1/1 -> Unit Delay2/1
  Unit Delay2/1 -> Detect Increase/1
  Unit Delay4/1 -> Unit Delay5/1
  Unit Delay5/1 -> Unit Delay6/1
  Unit Delay6/1 -> MCPInitialized/1
  Unit Delay7/1 -> Unit Delay4/1

== system ENV_old/Subsystem1 ==
  Detect Increase : simulink/Logic and Bit Operations/Detect Increase  vinit=0.0  OutDataTypeStr=boolean
  Initialize : Subsystem  TreatAsAtomicUnit=on
  MCPInit : Subsystem  TreatAsAtomicUnit=on
  Step1 : Step
  Step2 : Step
  Unit Delay : UnitDelay  SampleTime=-1  HasFrameUpgradeWarning=on
  MCPInitialized : Outport
  wires:
  Step1/1 -> Detect Increase/1
  Unit Delay/1 -> Initialize/Enable
  Detect Increase/1 -> MCPInit/Enable
  Step2/1 -> Unit Delay/1
  Initialize/1(MCPInitialized) -> MCPInitialized/1

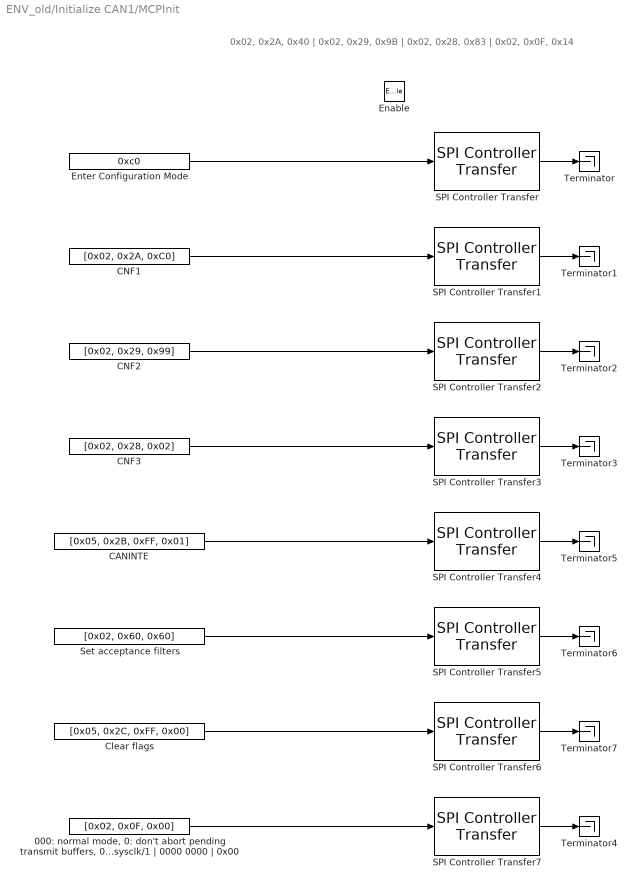
== system ENV_old/Initialize CAN1/MCPInit ==
  note: 0x02, 0x2A, 0x40 | 0x02, 0x29, 0x9B | 0x02, 0x28, 0x83 | 0x02, 0x0F, 0x14
  Enable : EnablePort
  " 000: normal mode, 0: don't abort pending transmit buffers, 0: one-shot disabled, 0: CLKOUT disabled, 00: sysclk/1 | 0000 0000 | 0x00" : Constant  Value=[0x02, 0x0F, 0x00]  OutDataTypeStr=uint8
  CANINTE : Constant  Value=[0x05, 0x2B, 0xFF, 0x01]  OutDataTypeStr=uint8
  CNF1 : Constant  Value=[0x02, 0x2A, 0xC0]  OutDataTypeStr=uint8
  CNF2 : Constant  Value=[0x02, 0x29, 0x99]  OutDataTypeStr=uint8
  CNF3 : Constant  Value=[0x02, 0x28, 0x02]  OutDataTypeStr=uint8
  Clear flags : Constant  Value=[0x05, 0x2C, 0xFF, 0x00]  OutDataTypeStr=uint8
  Enter Configuration Mode : Constant  Value=0xc0  OutDataTypeStr=uint8
  SPI Controller Transfer : stm32blockslib/SPI Controller Transfer  Priority=1  SPIModuleSelect=SPI1  ClockPolarity=Low  ClockPhase=1 Edge  SPIModule=uint32(0)  Mode=Master  BusSpeed=uint32(1000000)  FirstBitToTransfer=Most significant bit (MSB)  ClockMode=0  BlockFunction=Transfer  EnableRegisterAddress=off  RegisterAddress=0  OutputDataType=uint8  OutputDataLength=1  OutputStatus=off  BlockingMode=on  Timeout=0.01  DataBits=8  UseCustomSSPin=Explicit GPIO calls  ActiveLowSSPin=Active low  Port_Select=GPIOB  Pin=1
      settings: LibrarySourceBlock=stm32h7xxblockslib/SPI Controller Transfer
  SPI Controller Transfer1 : stm32blockslib/SPI Controller Transfer  Priority=2  SPIModuleSelect=SPI1  ClockPolarity=Low  ClockPhase=1 Edge  SPIModule=uint32(0)  Mode=Master  BusSpeed=uint32(1000000)  FirstBitToTransfer=Most significant bit (MSB)  ClockMode=0  BlockFunction=Transfer  EnableRegisterAddress=off  RegisterAddress=0  OutputDataType=uint8  OutputDataLength=1  OutputStatus=off  BlockingMode=on  Timeout=0.01  DataBits=8  UseCustomSSPin=Explicit GPIO calls  ActiveLowSSPin=Active low  Port_Select=GPIOB  Pin=1
      settings: LibrarySourceBlock=stm32h7xxblockslib/SPI Controller Transfer
  SPI Controller Transfer2 : stm32blockslib/SPI Controller Transfer  Priority=3  SPIModuleSelect=SPI1  ClockPolarity=Low  ClockPhase=1 Edge  SPIModule=uint32(0)  Mode=Master  BusSpeed=uint32(1000000)  FirstBitToTransfer=Most significant bit (MSB)  ClockMode=0  BlockFunction=Transfer  EnableRegisterAddress=off  RegisterAddress=0  OutputDataType=uint8  OutputDataLength=1  OutputStatus=off  BlockingMode=on  Timeout=0.01  DataBits=8  UseCustomSSPin=Explicit GPIO calls  ActiveLowSSPin=Active low  Port_Select=GPIOB  Pin=1
      settings: LibrarySourceBlock=stm32h7xxblockslib/SPI Controller Transfer
  SPI Controller Transfer3 : stm32blockslib/SPI Controller Transfer  Priority=4  SPIModuleSelect=SPI1  ClockPolarity=Low  ClockPhase=1 Edge  SPIModule=uint32(0)  Mode=Master  BusSpeed=uint32(1000000)  FirstBitToTransfer=Most significant bit (MSB)  ClockMode=0  BlockFunction=Transfer  EnableRegisterAddress=off  RegisterAddress=0  OutputDataType=uint8  OutputDataLength=1  OutputStatus=off  BlockingMode=on  Timeout=0.01  DataBits=8  UseCustomSSPin=Explicit GPIO calls  ActiveLowSSPin=Active low  Port_Select=GPIOB  Pin=1
      settings: LibrarySourceBlock=stm32h7xxblockslib/SPI Controller Transfer
  SPI Controller Transfer4 : stm32blockslib/SPI Controller Transfer  Priority=5  SPIModuleSelect=SPI1  ClockPolarity=Low  ClockPhase=1 Edge  SPIModule=uint32(0)  Mode=Master  BusSpeed=uint32(1000000)  FirstBitToTransfer=Most significant bit (MSB)  ClockMode=0  BlockFunction=Transfer  EnableRegisterAddress=off  RegisterAddress=0  OutputDataType=uint8  OutputDataLength=1  OutputStatus=off  BlockingMode=on  Timeout=0.01  DataBits=8  UseCustomSSPin=Explicit GPIO calls  ActiveLowSSPin=Active low  Port_Select=GPIOB  Pin=1
      settings: LibrarySourceBlock=stm32h7xxblockslib/SPI Controller Transfer
  SPI Controller Transfer5 : stm32blockslib/SPI Controller Transfer  Priority=6  SPIModuleSelect=SPI1  ClockPolarity=Low  ClockPhase=1 Edge  SPIModule=uint32(0)  Mode=Master  BusSpeed=uint32(1000000)  FirstBitToTransfer=Most significant bit (MSB)  ClockMode=0  BlockFunction=Transfer  EnableRegisterAddress=off  RegisterAddress=0  OutputDataType=uint8  OutputDataLength=1  OutputStatus=off  BlockingMode=on  Timeout=0.01  DataBits=8  UseCustomSSPin=Explicit GPIO calls  ActiveLowSSPin=Active low  Port_Select=GPIOB  Pin=1
      settings: LibrarySourceBlock=stm32h7xxblockslib/SPI Controller Transfer
  SPI Controller Transfer6 : stm32blockslib/SPI Controller Transfer  Priority=7  SPIModuleSelect=SPI1  ClockPolarity=Low  ClockPhase=1 Edge  SPIModule=uint32(0)  Mode=Master  BusSpeed=uint32(1000000)  FirstBitToTransfer=Most significant bit (MSB)  ClockMode=0  BlockFunction=Transfer  EnableRegisterAddress=off  RegisterAddress=0  OutputDataType=uint8  OutputDataLength=1  OutputStatus=off  BlockingMode=on  Timeout=0.01  DataBits=8  UseCustomSSPin=Explicit GPIO calls  ActiveLowSSPin=Active low  Port_Select=GPIOB  Pin=1
      settings: LibrarySourceBlock=stm32h7xxblockslib/SPI Controller Transfer
  SPI Controller Transfer7 : stm32blockslib/SPI Controller Transfer  Priority=8  SPIModuleSelect=SPI1  ClockPolarity=Low  ClockPhase=1 Edge  SPIModule=uint32(0)  Mode=Master  BusSpeed=uint32(1000000)  FirstBitToTransfer=Most significant bit (MSB)  ClockMode=0  BlockFunction=Transfer  EnableRegisterAddress=off  RegisterAddress=0  OutputDataType=uint8  OutputDataLength=1  OutputStatus=off  BlockingMode=on  Timeout=0.01  DataBits=8  UseCustomSSPin=Explicit GPIO calls  ActiveLowSSPin=Active low  Port_Select=GPIOB  Pin=1
      settings: LibrarySourceBlock=stm32h7xxblockslib/SPI Controller Transfer
  Set acceptance filters : Constant  Value=[0x02, 0x60, 0x60]  OutDataTypeStr=uint8
  Terminator{,1..7} (8 alike) : Terminator
  wires:
  SPI Controller Transfer6/1 -> Terminator7/1
  CNF3/1 -> SPI Controller Transfer3/1
  SPI Controller Transfer5/1 -> Terminator6/1
  CNF2/1 -> SPI Controller Transfer2/1
  CNF1/1 -> SPI Controller Transfer1/1
  SPI Controller Transfer3/1 -> Terminator3/1
  SPI Controller Transfer1/1 -> Terminator1/1
  Clear flags/1 -> SPI Controller Transfer6/1
  SPI Controller Transfer4/1 -> Terminator5/1
  SPI Controller Transfer2/1 -> Terminator2/1
  " 000: normal mode, 0: don't abort pending transmit buffers, 0: one-shot disabled, 0: CLKOUT disabled, 00: sysclk/1 | 0000 0000 | 0x00"/1 -> SPI Controller Transfer7/1
  SPI Controller Transfer7/1 -> Terminator4/1
  CANINTE/1 -> SPI Controller Transfer4/1
  Set acceptance filters/1 -> SPI Controller Transfer5/1
  Enter Configuration Mode/1 -> SPI Controller Transfer/1
  SPI Controller Transfer/1 -> Terminator/1

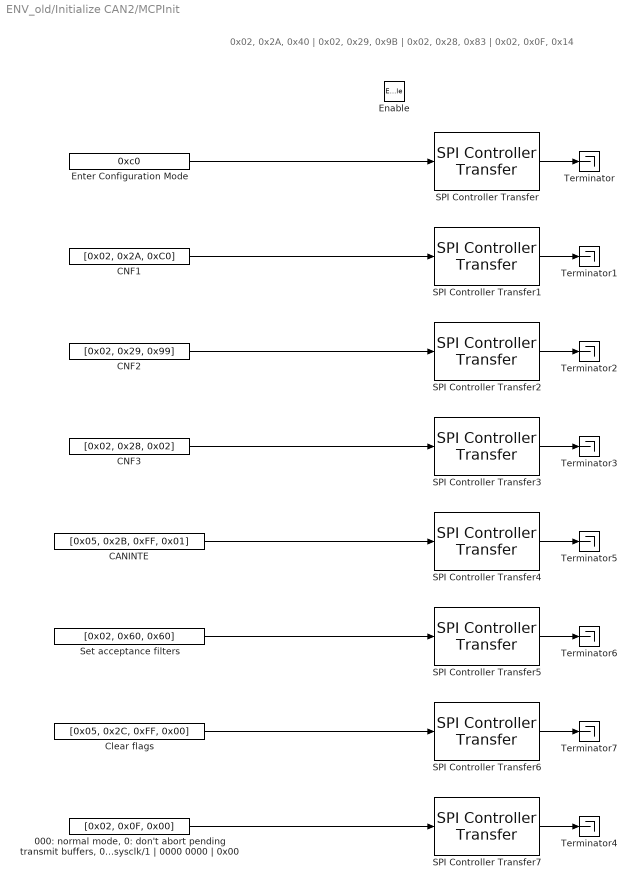
== system ENV_old/Initialize CAN2/MCPInit ==
  note: 0x02, 0x2A, 0x40 | 0x02, 0x29, 0x9B | 0x02, 0x28, 0x83 | 0x02, 0x0F, 0x14
  Enable : EnablePort
  " 000: normal mode, 0: don't abort pending transmit buffers, 0: one-shot disabled, 0: CLKOUT disabled, 00: sysclk/1 | 0000 0000 | 0x00" : Constant  Value=[0x02, 0x0F, 0x00]  OutDataTypeStr=uint8
  CANINTE : Constant  Value=[0x05, 0x2B, 0xFF, 0x01]  OutDataTypeStr=uint8
  CNF1 : Constant  Value=[0x02, 0x2A, 0xC0]  OutDataTypeStr=uint8
  CNF2 : Constant  Value=[0x02, 0x29, 0x99]  OutDataTypeStr=uint8
  CNF3 : Constant  Value=[0x02, 0x28, 0x02]  OutDataTypeStr=uint8
  Clear flags : Constant  Value=[0x05, 0x2C, 0xFF, 0x00]  OutDataTypeStr=uint8
  Enter Configuration Mode : Constant  Value=0xc0  OutDataTypeStr=uint8
  SPI Controller Transfer : stm32blockslib/SPI Controller Transfer  Priority=1  SPIModuleSelect=SPI1  ClockPolarity=Low  ClockPhase=1 Edge  SPIModule=uint32(0)  Mode=Master  BusSpeed=uint32(1000000)  FirstBitToTransfer=Most significant bit (MSB)  ClockMode=0  BlockFunction=Transfer  EnableRegisterAddress=off  RegisterAddress=0  OutputDataType=uint8  OutputDataLength=1  OutputStatus=off  BlockingMode=on  Timeout=0.01  DataBits=8  UseCustomSSPin=Explicit GPIO calls  ActiveLowSSPin=Active low  Port_Select=GPIOC  Pin=10
      settings: LibrarySourceBlock=stm32h7xxblockslib/SPI Controller Transfer
  SPI Controller Transfer1 : stm32blockslib/SPI Controller Transfer  Priority=2  SPIModuleSelect=SPI1  ClockPolarity=Low  ClockPhase=1 Edge  SPIModule=uint32(0)  Mode=Master  BusSpeed=uint32(1000000)  FirstBitToTransfer=Most significant bit (MSB)  ClockMode=0  BlockFunction=Transfer  EnableRegisterAddress=off  RegisterAddress=0  OutputDataType=uint8  OutputDataLength=1  OutputStatus=off  BlockingMode=on  Timeout=0.01  DataBits=8  UseCustomSSPin=Explicit GPIO calls  ActiveLowSSPin=Active low  Port_Select=GPIOC  Pin=10
      settings: LibrarySourceBlock=stm32h7xxblockslib/SPI Controller Transfer
  SPI Controller Transfer2 : stm32blockslib/SPI Controller Transfer  Priority=3  SPIModuleSelect=SPI1  ClockPolarity=Low  ClockPhase=1 Edge  SPIModule=uint32(0)  Mode=Master  BusSpeed=uint32(1000000)  FirstBitToTransfer=Most significant bit (MSB)  ClockMode=0  BlockFunction=Transfer  EnableRegisterAddress=off  RegisterAddress=0  OutputDataType=uint8  OutputDataLength=1  OutputStatus=off  BlockingMode=on  Timeout=0.01  DataBits=8  UseCustomSSPin=Explicit GPIO calls  ActiveLowSSPin=Active low  Port_Select=GPIOC  Pin=10
      settings: LibrarySourceBlock=stm32h7xxblockslib/SPI Controller Transfer
  SPI Controller Transfer3 : stm32blockslib/SPI Controller Transfer  Priority=4  SPIModuleSelect=SPI1  ClockPolarity=Low  ClockPhase=1 Edge  SPIModule=uint32(0)  Mode=Master  BusSpeed=uint32(1000000)  FirstBitToTransfer=Most significant bit (MSB)  ClockMode=0  BlockFunction=Transfer  EnableRegisterAddress=off  RegisterAddress=0  OutputDataType=uint8  OutputDataLength=1  OutputStatus=off  BlockingMode=on  Timeout=0.01  DataBits=8  UseCustomSSPin=Explicit GPIO calls  ActiveLowSSPin=Active low  Port_Select=GPIOC  Pin=10
      settings: LibrarySourceBlock=stm32h7xxblockslib/SPI Controller Transfer
  SPI Controller Transfer4 : stm32blockslib/SPI Controller Transfer  Priority=5  SPIModuleSelect=SPI1  ClockPolarity=Low  ClockPhase=1 Edge  SPIModule=uint32(0)  Mode=Master  BusSpeed=uint32(1000000)  FirstBitToTransfer=Most significant bit (MSB)  ClockMode=0  BlockFunction=Transfer  EnableRegisterAddress=off  RegisterAddress=0  OutputDataType=uint8  OutputDataLength=1  OutputStatus=off  BlockingMode=on  Timeout=0.01  DataBits=8  UseCustomSSPin=Explicit GPIO calls  ActiveLowSSPin=Active low  Port_Select=GPIOC  Pin=10
      settings: LibrarySourceBlock=stm32h7xxblockslib/SPI Controller Transfer
  SPI Controller Transfer5 : stm32blockslib/SPI Controller Transfer  Priority=6  SPIModuleSelect=SPI1  ClockPolarity=Low  ClockPhase=1 Edge  SPIModule=uint32(0)  Mode=Master  BusSpeed=uint32(1000000)  FirstBitToTransfer=Most significant bit (MSB)  ClockMode=0  BlockFunction=Transfer  EnableRegisterAddress=off  RegisterAddress=0  OutputDataType=uint8  OutputDataLength=1  OutputStatus=off  BlockingMode=on  Timeout=0.01  DataBits=8  UseCustomSSPin=Explicit GPIO calls  ActiveLowSSPin=Active low  Port_Select=GPIOC  Pin=10
      settings: LibrarySourceBlock=stm32h7xxblockslib/SPI Controller Transfer
  SPI Controller Transfer6 : stm32blockslib/SPI Controller Transfer  Priority=7  SPIModuleSelect=SPI1  ClockPolarity=Low  ClockPhase=1 Edge  SPIModule=uint32(0)  Mode=Master  BusSpeed=uint32(1000000)  FirstBitToTransfer=Most significant bit (MSB)  ClockMode=0  BlockFunction=Transfer  EnableRegisterAddress=off  RegisterAddress=0  OutputDataType=uint8  OutputDataLength=1  OutputStatus=off  BlockingMode=on  Timeout=0.01  DataBits=8  UseCustomSSPin=Explicit GPIO calls  ActiveLowSSPin=Active low  Port_Select=GPIOC  Pin=10
      settings: LibrarySourceBlock=stm32h7xxblockslib/SPI Controller Transfer
  SPI Controller Transfer7 : stm32blockslib/SPI Controller Transfer  Priority=8  SPIModuleSelect=SPI1  ClockPolarity=Low  ClockPhase=1 Edge  SPIModule=uint32(0)  Mode=Master  BusSpeed=uint32(1000000)  FirstBitToTransfer=Most significant bit (MSB)  ClockMode=0  BlockFunction=Transfer  EnableRegisterAddress=off  RegisterAddress=0  OutputDataType=uint8  OutputDataLength=1  OutputStatus=off  BlockingMode=on  Timeout=0.01  DataBits=8  UseCustomSSPin=Explicit GPIO calls  ActiveLowSSPin=Active low  Port_Select=GPIOC  Pin=10
      settings: LibrarySourceBlock=stm32h7xxblockslib/SPI Controller Transfer
  Set acceptance filters : Constant  Value=[0x02, 0x60, 0x60]  OutDataTypeStr=uint8
  Terminator{,1..7} (8 alike) : Terminator
  wires:
  SPI Controller Transfer6/1 -> Terminator7/1
  CNF3/1 -> SPI Controller Transfer3/1
  SPI Controller Transfer5/1 -> Terminator6/1
  CNF2/1 -> SPI Controller Transfer2/1
  CNF1/1 -> SPI Controller Transfer1/1
  SPI Controller Transfer3/1 -> Terminator3/1
  SPI Controller Transfer1/1 -> Terminator1/1
  Clear flags/1 -> SPI Controller Transfer6/1
  SPI Controller Transfer4/1 -> Terminator5/1
  SPI Controller Transfer2/1 -> Terminator2/1
  " 000: normal mode, 0: don't abort pending transmit buffers, 0: one-shot disabled, 0: CLKOUT disabled, 00: sysclk/1 | 0000 0000 | 0x00"/1 -> SPI Controller Transfer7/1
  SPI Controller Transfer7/1 -> Terminator4/1
  CANINTE/1 -> SPI Controller Transfer4/1
  Set acceptance filters/1 -> SPI Controller Transfer5/1
  Enter Configuration Mode/1 -> SPI Controller Transfer/1
  SPI Controller Transfer/1 -> Terminator/1
